simulink model "Lab_6_1"  (R2016a)
settings: Solver=VariableStepAuto  StartTime=0.0  StopTime=10.0  RelTol=1e-3
settings Model: Creator=Asus  LastModifiedBy=Asus

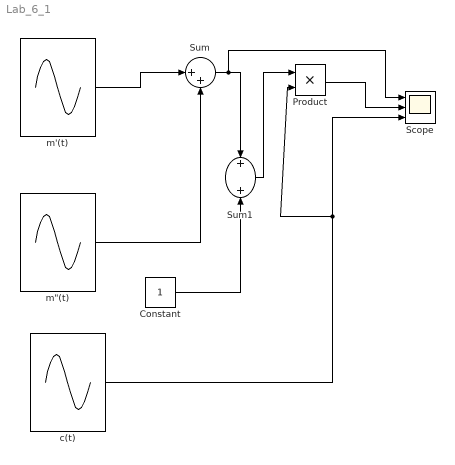
== system Lab_6_1 ==
  Constant : Constant
  Product : Product
  Scope : Scope  NumInputPorts=3
  Sum : Sum  Inputs=|++
  Sum1 : Sum
  c(t) : Sin  Frequency=2*pi*50  Phase=pi/2  SampleTime=1/5000
  "m\"(t)" : Sin  Amplitude=3  Frequency=2*pi*6  Phase=pi/2  SampleTime=1/5000
  m'(t) : Sin  Amplitude=2  Frequency=2*pi*4  SampleTime=1/5000
  wires:
  m'(t)/1 -> Sum/1
  "m\"(t)"/1 -> Sum/2
  Sum1/1 -> Product/1
  Constant/1 -> Sum1/2
  c(t)/1 -> Scope/3, Product/2
  Product/1 -> Scope/2
  Sum/1 -> Scope/1, Sum1/1
